simulink model "sixoneone"  (R2020a)
settings: Solver=VariableStepAuto  StartTime=0.0  StopTime=10.0  RelTol=1e-3
values from neighbouring files (symbols this model uses):
  B1 = [1 0;1 0;1 1;1 1]    [sixone.m]
  U1 = [u1,u2]    [sixone.m]
  U2 = [u3,u4]    [sixone.m]
undefined symbols (not defined in the file or in its folder): A, B, C
settings Model: Creator=wyton  LastModifiedBy=wyton

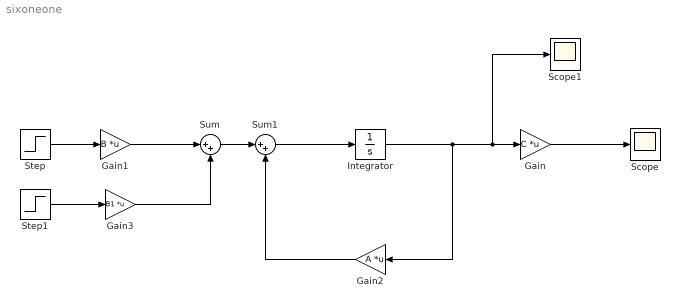
== system sixoneone ==
  Gain : Gain  Gain=C  Multiplication=Matrix(K*u)
  Gain1 : Gain  Gain=B  Multiplication=Matrix(K*u)
  Gain2 : Gain  Gain=A  Multiplication=Matrix(K*u)
  Gain3 : Gain  Gain=B1  Multiplication=Matrix(K*u)
  Integrator : Integrator
  Scope : Scope
  Scope1 : Scope
  Step : Step  Before=[0;0]  After=U1  SampleTime=0
  Step1 : Step  After=U2  SampleTime=0
  Sum : Sum  Inputs=|++
  Sum1 : Sum  Inputs=|++
  wires:
  Gain/1 -> Scope/1
  Integrator/1 -> Gain2/1, Scope1/1, Gain/1
  Gain1/1 -> Sum/1
  Gain3/1 -> Sum/2
  Sum/1 -> Sum1/1
  Gain2/1 -> Sum1/2
  Step1/1 -> Gain3/1
  Step/1 -> Gain1/1
  Sum1/1 -> Integrator/1
